simulink model "Modello_con_subsystem"  (Simulink 7.8)
settings: Solver=ode45  StartTime=0.0  StopTime=1500  RelTol=1e-3
values from neighbouring files (symbols this model uses):
  A = [A_longitudinale, zeros(4,4) ; zeros(4,4) , A_laterale]    [Matlab_6gdl_in_s.m]
  B = [B_longitudinale ; B_laterale]    [Matlab_6gdl_in_s.m]
  C = eye(8)    [Matlab_6gdl_in_s.m]
  D = zeros(8,1)    [Matlab_6gdl_in_s.m]
undefined symbols (not defined in the file or in its folder): dimensionalizzazione
settings Model: Creator=Adriano  LastModifiedBy=Adriano
settings DataIOCC: LimitDataPoints=off

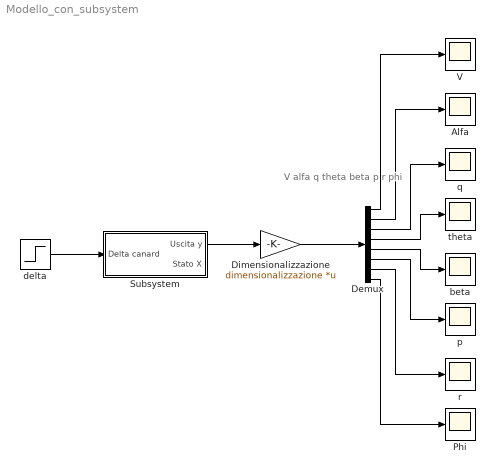
== system Modello_con_subsystem ==
  note: V
      | alfa
      | q
      | theta
      | beta
      | p
      | r
      | phi
  Alfa : Scope
  Demux : Demux  Outputs=8
  Dimensionalizzazione : Gain  Gain=dimensionalizzazione  Multiplication=Matrix(K*u)
  Phi : Scope
      settings: SaveName=ScopeData7
  Subsystem : Subsystem
  V : Scope
  beta : Scope
      settings: TimeRange=50  YMin=-0.01  YMax=0.06000000000000001  SaveName=ScopeData4
  delta : Step  Time=500  After=0.17  SampleTime=0
  p : Scope
      settings: SaveName=ScopeData5
  q : Scope
      settings: TimeRange=500  YMin=-1  YMax=1  SaveName=ScopeData2
  r : Scope
      settings: SaveName=ScopeData6
  theta : Scope
      settings: SaveName=ScopeData3
  wires:
  Subsystem/1(Uscita y) -> Dimensionalizzazione/1
  Dimensionalizzazione/1 -> Demux/1
  Demux/1 -> V/1
  Demux/2 -> Alfa/1
  Demux/3 -> q/1
  Demux/4 -> theta/1
  Demux/5 -> beta/1
  Demux/6 -> p/1
  Demux/7 -> r/1
  Demux/8 -> Phi/1
  delta/1 -> Subsystem/1(Delta canard)

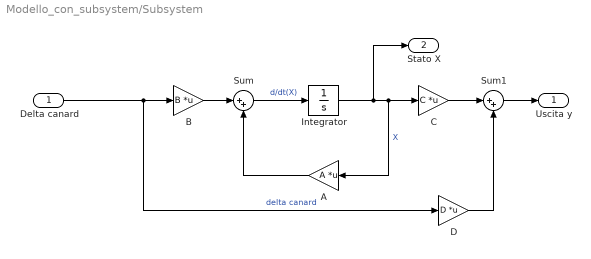
== system Modello_con_subsystem/Subsystem ==
  Delta canard : Inport
  A : Gain  Gain=A  Multiplication=Matrix(K*u) (u vector)
  B : Gain  Gain=B  Multiplication=Matrix(K*u) (u vector)
  C : Gain  Gain=C  Multiplication=Matrix(K*u) (u vector)
  D : Gain  Gain=D  Multiplication=Matrix(K*u) (u vector)
  Integrator : Integrator
  Sum : Sum  Inputs=|++
  Sum1 : Sum  Inputs=|++
  Uscita y : Outport
  Stato X : Outport  Port=2
  wires:
  Integrator/1 -> C/1, A/1, Stato X/1  "X"
  A/1 -> Sum/2
  Sum/1 -> Integrator/1  "d/dt(X)"
  B/1 -> Sum/1
  Delta canard/1 -> B/1, D/1  "delta canard"
  C/1 -> Sum1/1
  D/1 -> Sum1/2
  Sum1/1 -> Uscita y/1
